simulink library "Economy_Ecology"  (Simulink 8.8)
settings: Solver=ode45  StartTime=0.0  StopTime=10.0  RelTol=1e-3  EnableMultiTasking=on
libraries: carnot x1
settings Model: Creator=lena.frank  LastModifiedBy=User

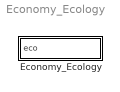
== system Economy_Ecology ==
  Economy_Ecology : Subsystem  mask(economy_ecology){}
      mask help: Calculates massflow, costs, exhaust gas etc.
      mask Help: web(fullfile(path_carnot('help'),'economy_ecology.html'),'-helpbrowser')

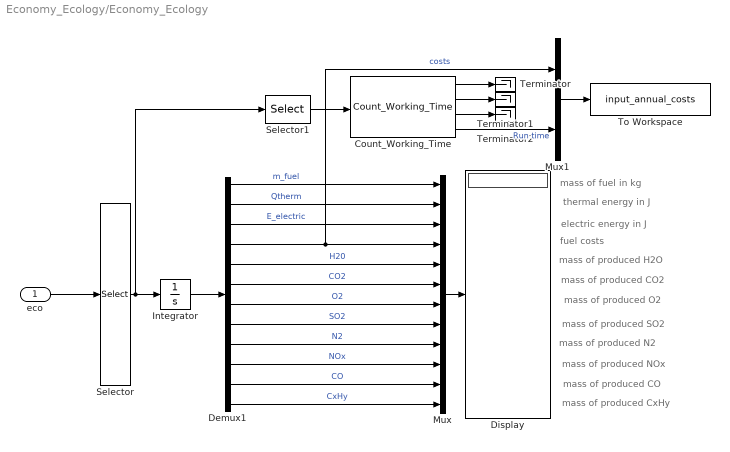
== system Economy_Ecology/Economy_Ecology ==
  note: mass of produced CxHy
  note: mass of produced CO
  note: mass of produced NOx
  note: mass of produced N2
  note: mass of produced SO2
  note: mass of produced O2
  note: mass of produced CO2
  note: mass of produced H2O
  note: fuel costs
  note: electric energy in J
  note: thermal energy in J
  note: mass of fuel in kg
  eco : Inport
  Count_Working_Time : carnot/Toolbox/Count_Working_Time
  Demux1 : Demux  Outputs=12
  Display : Display
  Integrator : Integrator
  Mux : Mux  Inputs=12
  Mux1 : Mux  Inputs=2
  Selector : Selector  InputPortWidth=16  IndexOptions=Index vector (dialog)  Indices=[3 5:15]  OutputSizes=1
  Selector1 : Selector  InputPortWidth=12  IndexOptions=Index vector (dialog)  Indices=[1]  OutputSizes=1
  Terminator : Terminator
  Terminator1 : Terminator
  Terminator2 : Terminator
  To Workspace : ToWorkspace  VariableName=input_annual_costs  SampleTime=-1
      settings: MaxDataPoints=1
  wires:
  Demux1/8 -> Mux/8  "SO2"
  Demux1/5 -> Mux/5  "H20"
  Demux1/7 -> Mux/7  "O2"
  eco/1 -> Selector/1
  Integrator/1 -> Demux1/1
  Demux1/6 -> Mux/6  "CO2"
  Demux1/9 -> Mux/9  "N2"
  Demux1/12 -> Mux/12  "CxHy"
  Demux1/11 -> Mux/11  "CO"
  Demux1/10 -> Mux/10  "NOx"
  Demux1/2 -> Mux/2  "Qtherm"
  Demux1/3 -> Mux/3  "E_electric"
  Mux/1 -> Display/1
  Mux1/1 -> To Workspace/1
  Selector/1 -> Integrator/1, Selector1/1
  Selector1/1 -> Count_Working_Time/1
  Demux1/1 -> Mux/1  "m_fuel"
  Demux1/4 -> Mux/4, Mux1/1  "costs"
  Count_Working_Time/4 -> Mux1/2  "Run time"
  Count_Working_Time/1 -> Terminator/1
  Count_Working_Time/2 -> Terminator1/1
  Count_Working_Time/3 -> Terminator2/1
